simulink model "rtwdemo_lct_ndarray"  (Simulink 7.6)
settings: Solver=ode5  StartTime=0.0  StopTime=30  RelTol=1e-3  SampleTimeConstraint=STIndependent
libraries: rtwdemowidgets x2
Description:
  | Inherited Signal Dimensions
settings Model: Creator=The MathWorks Inc.  ExtModeAutoUpdateStatusClock=off
settings DataIOCC: SignalLoggingName=logsOut
settings OptimizationCC: InlineParams=on  InlineInvariantSignals=on  EfficientFloat2IntCast=on  EfficientMapNaN2IntZero=off
settings DebuggingCC: CheckExecutionContextPreStartOutputMsg=on  CheckExecutionContextRuntimeOutputMsg=on  SolverPrmCheckMsg=none  BusObjectLabelMismatch=error  StrictBusMsg=ErrorOnBusTreatedAsVector
settings HardwareCC: ProdIntDivRoundTo=Zero  ProdEndianess=LittleEndian  ProdHWDeviceType=Generic->32-bit Embedded Processor  TargetHWDeviceType=Generic->32-bit Embedded Processor
settings ModelReferenceCC: UpdateModelReferenceTargets=IfOutOfDate
settings RTWCC: TLCOptions=-p0 -aWarnNonSaturatedBlocks=0  GenerateReport=on  RTWVerbose=off  ProcessScript=grt_make_rtw_hook  LaunchReport=on
settings CodeAppCC: ForceParamTrailComments=on
settings GRTTargetCC: TargetFcnLib=ansi_tfl_tmw.mat

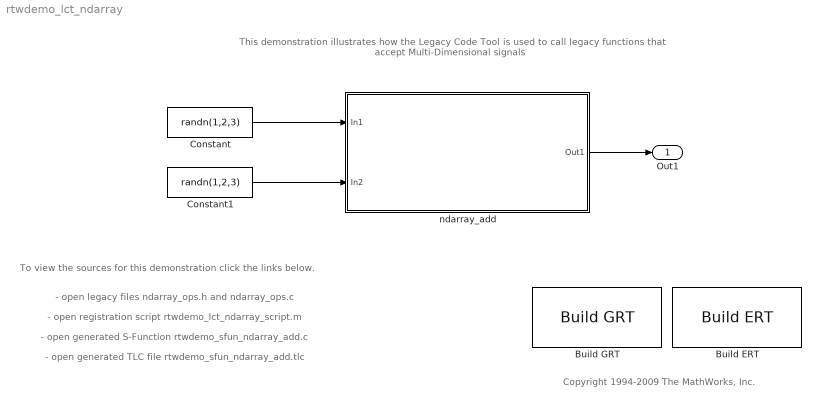
== system rtwdemo_lct_ndarray ==
  note: This demonstration illustrates how the Legacy Code Tool is used to
      | call legacy functions that accept Multi-Dimensional signals
  note: - open legacy files ndarray_ops.h and ndarray_ops.c
  note: To view the sources for this demonstration
      | click the links below.
  note: - open registration script rtwdemo_lct_ndarray_script.m
  note: - open generated S-Function rtwdemo_sfun_ndarray_add.c
  note: Copyright 1994-2009 The MathWorks, Inc.
  note: - open generated TLC file rtwdemo_sfun_ndarray_add.tlc
  Build ERT : rtwdemowidgets/Build ERT  SystemSampleTime=-1  attrib_overrides={}
  Build GRT : rtwdemowidgets/Build GRT  SystemSampleTime=-1  attrib_overrides={}
  Constant : Constant  Value=randn(1,2,3)  OutDataTypeStr=double
  Constant1 : Constant  Value=randn(1,2,3)  OutDataTypeStr=double
  ndarray_add : Subsystem
  Out1 : Outport
  wires:
  ndarray_add/1(Out1) -> Out1/1
  Constant/1 -> ndarray_add/1(In1)
  Constant1/1 -> ndarray_add/2(In2)

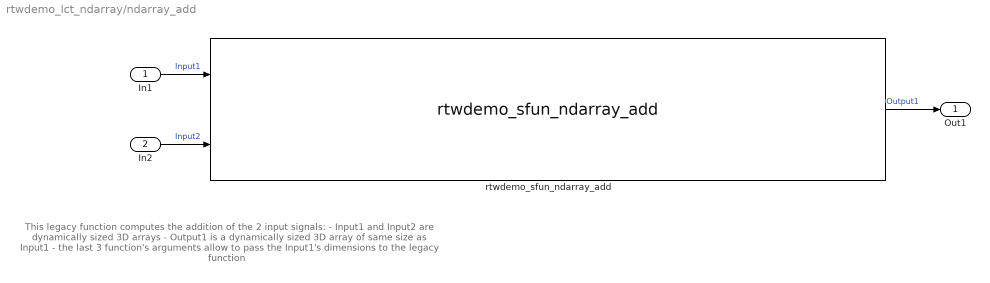
== system rtwdemo_lct_ndarray/ndarray_add ==
  note: This legacy function computes the addition of the 2 input signals:
      |    - Input1 and Input2 are dynamically sized 3D arrays
      |    - Output1 is a dynamically sized 3D array of same size as Input1
      |    - the last 3 function's arguments allow to pass the Input1's dimensions to the legacy function
  In1 : Inport
  In2 : Inport  Port=2
  rtwdemo_sfun_ndarray_add : S-Function  FunctionName=rtwdemo_sfun_ndarray_add  EnableBusSupport=off  mask(Legacy Function){SFunctionSpec=void array3d_add(double y1[size(u1,1)][size(u1,2)][size(u1,3)], double u1[][][], double u2[][][], int32 size(u1,1), int32 size(u1,2), int32 size(u1,3)), ShowSpec=on}
      mask prompts: ShowSpec "Display function specification"
      mask help:
      | This block allows you to call the legacy functions specified by the following Legacy Code Tool definition:
      | def.SFunctionName = 'rtwdemo_sfun_ndarray_add';
      | def.OutputFcnSpec = 'void array3d_add(double y1[size(u1,1)][size(u1,2)][size(u1,3)], double u1[][][], double u2[][][], int32 size(u1,1), int32 size(u1,2), int32 size(u1,3))';
      | def.HeaderFiles = {'ndarray_ops.h'};
      | def.SourceFiles = {'ndarray_ops.c'};
      | def.IncPaths = {'sldemo_lct_src'};
      | def.SrcPaths = {'sldemo_lct_src'};
      mask Help: <p>This block was generated automatically by the Legacy Code Tool. For detailed help on this tool, call<a href="matlab:legacy_code('help')"> legacy_code('help')</a>.</p>
      mask CallbackString:
      | |if strcmp(get_param(gcbh, 'ShowSpec'), 'on')
      |   set_param(gcbh, 'MaskDisplay', sprintf('fprintf(''%s'');', get_param(gcbh, 'SFunctionSpec')));
      | else
      |   set_param(gcbh, 'MaskDisplay', sprintf('fprintf(''%s'');', get_param(gcbh, 'FunctionName')));
      | end
      mask Display: fprintf('void array3d_add(double y1[size(u1,1)][size(u1,2)][size(u1,3)], double u1[][][], double u2[][][], int32 size(u1,1), int32 size(u1,2), int32 size(u1,3))');
  Out1 : Outport
  wires:
  In2/1 -> rtwdemo_sfun_ndarray_add/2  "Input2"
  rtwdemo_sfun_ndarray_add/1 -> Out1/1  "Output1"
  In1/1 -> rtwdemo_sfun_ndarray_add/1  "Input1"
